simulink model "Autoex"  (Simulink 6.5)
settings: Solver=ode23t  StartTime=0.0  StopTime=10  RelTol=1e-3
undefined symbols (not defined in the file): powergui
libraries: powerlib x10, powerlib_extras x1
settings Model: Creator=RS  LastModifiedBy=RS

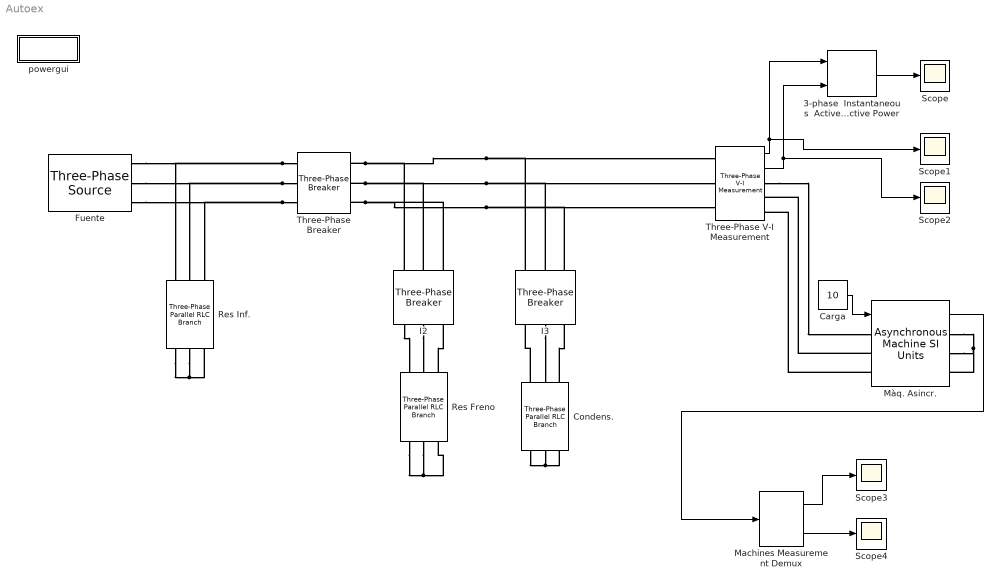
== system Autoex ==
  3-phase  Instantaneous  Active & Reactive Power : powerlib_extras/Measurements/3-phase  Instantaneous  Active & Reactive Power  DialogController=PMDialogs.PMDefaultMaskDlg  SystemSampleTime=-1
  Carga : Constant  Value=10  OutDataType=sfix(16)  ConRadixGroup=Use specified scaling  OutScaling=2^0  SampleTime=inf  FramePeriod=inf
  Condens. : powerlib/Elements/Three-Phase Parallel RLC Branch  Orientation=down  DialogController=PMDialogs.PMDefaultMaskDlg  PhysicalDomain=powersysdomain  SubClassName=unknown  LeftPortType=p1  RightPortType=p1  LConnTagsString=A|B|C  RConnTagsString=A|B|C  BranchType=C  Resistance=1  Inductance=1e-3  Capacitance=96.5e-6  Measurements=None
  Fuente : powerlib/Electrical Sources/Three-Phase Source  DialogController=PMDialogs.PMDefaultMaskDlg  SystemSampleTime=-1  Voltage=380  PhaseAngle=0  Frequency=50  InternalConnection=Yg  SpecifyImpedance=off  Resistance=0.0001  Inductance=0.0001  ShortCircuitLevel=100e6  BaseVoltage=25e3  XRratio=7
  I2 : powerlib/Elements/Three-Phase Breaker  Orientation=up  DialogController=PMDialogs.PMDefaultMaskDlg  SystemSampleTime=-1  InitialState=open  SwitchA=on  SwitchB=on  SwitchC=on  SwitchTimes=4  External=off  BreakerResistance=0.001  SnubberResistance=1e6  SnubberCapacitance=inf  Measurements=None
  I3 : powerlib/Elements/Three-Phase Breaker  Orientation=up  DialogController=PMDialogs.PMDefaultMaskDlg  SystemSampleTime=-1  InitialState=open  SwitchA=on  SwitchB=on  SwitchC=on  SwitchTimes=0  External=off  BreakerResistance=0.001  SnubberResistance=1e6  SnubberCapacitance=inf  Measurements=None
  Machines Measurement Demux : powerlib/Machines/Machines Measurement Demux  DialogController=PMDialogs.PMDefaultMaskDlg  SystemSampleTime=-1  machType=Asynchronous  ssm1=on  ssm2=on  ssm3=on  ssm4=on  ssm5=on  ssm6=on  sm1=off  sm2=off  sm3=off  sm4=off  sm5=off  sm6=off  sm7=off  sm8=on  sm9=off  sm10=off  sm11=off  sm115=off  sm12=off  sm13=off  sm14=off  asm1=off  asm2=off  asm3=off  asm4=off  asm5=off  asm6=off  asm7=off  asm8=off  asm9=on  asm10=on  asm11=off  pmsm1=on  pmsm2=on  pmsm3=on  pmsm4=off  pmsm5=on  pmsm6=on  pmsm7=on  lastType=1
  Màq. Asincr. : powerlib/Machines/Asynchronous Machine SI Units  DialogController=PMDialogs.PMDefaultMaskDlg  SystemSampleTime=-1  PresetModel=No  MechanicalLoad=Torque Tm  ShowDetailedParameters=on  RotorType=Wound  ReferenceFrame=Stationary  NominalParameters="[6.5*746   380   50]"  Stator="[0.63  0.00496]"  Rotor="[1.094   0.00496]"  Lm=0.105  Mechanical="[0.041   0   2]"  PolePairs=2  InitialConditions="[ 0,0   0,0,0   0,0,0 ]"  Units=1  LoadFlowParameters=0  SimulateSaturation=off  Saturation=[9.9249,19.6672,38.0377,51.3988,69.2824,105.1337,152.5532,214.2421,303.1917;230, 322, 414, 460, 506, 552, 598, 644, 690]
  Res Freno : powerlib/Elements/Three-Phase Parallel RLC Branch  Orientation=down  DialogController=PMDialogs.PMDefaultMaskDlg  PhysicalDomain=powersysdomain  SubClassName=unknown  LeftPortType=p1  RightPortType=p1  LConnTagsString=A|B|C  RConnTagsString=A|B|C  BranchType=R  Resistance=50  Inductance=1e-3  Capacitance=1e-6  Measurements=None
  Res Inf. : powerlib/Elements/Three-Phase Parallel RLC Branch  Orientation=down  DialogController=PMDialogs.PMDefaultMaskDlg  PhysicalDomain=powersysdomain  SubClassName=unknown  LeftPortType=p1  RightPortType=p1  LConnTagsString=A|B|C  RConnTagsString=A|B|C  BranchType=R  Resistance=1000000  Inductance=1e-3  Capacitance=1e-6  Measurements=None
  Scope{,1..4} (5 alike) : Scope
      Scope settings: MaxDataPoints=10000000  SampleInput=on  SampleTime=10e-6
      Scope1 settings: YMin=-1500  YMax=1500  MaxDataPoints=10000000  SampleInput=on  SampleTime=10e-6
      Scope2 settings: SaveName=ScopeData2  MaxDataPoints=10000000  SampleInput=on  SampleTime=10e-6
      Scope3 settings: SaveName=ScopeData3  MaxDataPoints=10000000  SampleInput=on  SampleTime=10e-6
      Scope4 settings: SaveName=ScopeData4  MaxDataPoints=10000000  SampleInput=on  SampleTime=10e-6
  Three-Phase V-I Measurement : powerlib/Measurements/Three-Phase V-I Measurement  DialogController=PMDialogs.PMDefaultMaskDlg  SystemSampleTime=-1  VoltageMeasurement=phase-to-ground  SetLabelV=off  LabelV=Vabc  Vpu=off  CurrentMeasurement=yes  SetLabelI=off  LabelI=Iabc  Ipu=off  Pbase=100e6  Vbase=500e3  OutputType=Complex  PhasorSimulation=off  PSBequivalent=0
  Three-Phase Breaker : powerlib/Elements/Three-Phase Breaker  DialogController=PMDialogs.PMDefaultMaskDlg  SystemSampleTime=-1  InitialState=closed  SwitchA=on  SwitchB=on  SwitchC=on  SwitchTimes=0  External=off  BreakerResistance=0.001  SnubberResistance=1e6  SnubberCapacitance=inf  Measurements=None
  powergui : Subsystem  AncestorBlock=powerlib/powergui  InitFcn=powergui( 'InitFcn_Callback' , gcb , 0 , [ ] );  mask(PSB option menu block){SimulationMode=Continuous, SampleTime=50e-6, echomessages=off, RestoreLinks=warning, x0status=blocks, Frange=[0:2:500], Ylog=off, Xlog=on, ShowGrid=off, save=off, variable=ZData, structure=, ZoomFFT=on, StartTime=0.0, cycles=1, DisplayStyle=1, fundamental=60, FreqAxis=off, MaxFrequency=1000, frequencyindice=50, frequencyindicesteady=1, RmsSteady=1, display=off, Ts=0, frequency=60, methode=off, HookPort=off, Interpol=off}
      mask prompts: SimulationMode "Simulation mode"; SampleTime "Sample time Ts (when simulation mode is Discrete) (s)"; echomessages "Echo  Messages"; RestoreLinks "Restore disabled links"; x0status "Initial electrical states status"; Frange "Impedance tool: Frequency Range"; Ylog "Impedance tool: Log impedance"; Xlog "Impedance tool: log Frequency"; ShowGrid "Impedance tool: grid"; save "Impedance tool: Save Data To Workspace"; variable "Impedance tool: Variable Name"; structure "Structure Name (PSBFFTSCOPE)"; ZoomFFT "ZoomFFT (PSBFFTSCOPE)"; StartTime "Start Time (PSBFFTSCOPE)"; cycles "Cycles (PSBFFTSCOPE)"; DisplayStyle "Display style (PSBFFTSCOPE)"; fundamental "Fundamental (PSBFFTSCOPE)"; FreqAxis "Frequency Axis (PSBFFTSCOPE)"; MaxFrequency "Max Frequency (PSBFFTSCOPE)"; frequencyindice "Load flow frequency (Hz)"; frequencyindicesteady "Frequency indice (STEADYSTATE)"; RmsSteady "RMS display (STEADYSTATE)"; display "Display Results"; Ts "OBSOLETE 1"; frequency "Phasor frequency (Hz)"; methode "Phasor simulation"; HookPort "Hook port"; Interpol "Interpolate"
      mask init:
      | powerlibroot = which('powersysdomain');
      | PSBroot = powerlibroot(1:end-16);
      | %
      | switch SimulationMode
      | 	case 1
      | 		message=sprintf('Continuous');
      | 	case 2
      |         SampleTimeeval=evalin('base',SampleTime,'NaN');
      |         if isnan(SampleTimeeval)
      |             message=sprintf('Warning !!,\nUndefined sample time');
      |         else
      |             message=sprintf('Discrete,\nTs = %.4g s.',SampleTimeeval);
      |         end
      | 	case 3
      | 		message=sprintf('Phasors');
      | end
      | if strcmp(bdroot,'powerlib')
      |   message='powergui';
      | end
      | power_initmask();
      settings: CopyFcn=powergui( 'Copy_Callback' , gcb , 0 , [ ] );  ModelCloseFcn=powergui( 'CloseButton_Callback' , gcb , [ ] , [ ] );  PreSaveFcn=powergui( 'CloseButton_Callback' , gcb , [ ] , [ ] );  NameChangeFcn=powergui( 'NameChangeFcn_Callback' , gcb , 0 , [ ] );
      settings: DeleteFcn=|
      | powergui( 'Copy_Callback' , gcb , 1 , [ ] );
      | powergui( 'CloseButton_Callback' , gcb , [ ] , [ ] );
      settings: OpenFcn=|
      | if (power_openblockproxy ('secondary'))
      | powergui(gcb,'PM')
      | end;
      mask Help: web(psbhelp)
      mask StyleString: popup(Continuous|Discrete|Phasor),edit,checkbox,popup(yes|warning|no),popup(blocks|steady|zero),edit,checkbox,checkbox,checkbox,checkbox,edit,edit,checkbox,edit,edit,edit,edit,checkbox,edit,edit,edit,edit,checkbox,edit,edit,checkbox,checkbox,checkbox
      mask CallbackString: ||||||||||||||||||||||||||powergui('HookPort',[],[],gcb);|
      mask Display: disp(message)
  wires:
  Three-Phase V-I Measurement/1 -> 3-phase  Instantaneous  Active & Reactive Power/1, Scope1/1
  Three-Phase V-I Measurement/2 -> 3-phase  Instantaneous  Active & Reactive Power/2, Scope2/1
  Màq. Asincr./1 -> Machines Measurement Demux/1
  Carga/1 -> Màq. Asincr./1
  3-phase  Instantaneous  Active & Reactive Power/1 -> Scope/1
  Machines Measurement Demux/1 -> Scope3/1
  Machines Measurement Demux/2 -> Scope4/1
  connections:
  Three-Phase Breaker/RConn2 -- I2/RConn2 -- Three-Phase V-I Measurement/LConn2 -- I3/RConn2
  Three-Phase Breaker/RConn1 -- I2/RConn1 -- Three-Phase V-I Measurement/LConn1 -- I3/RConn1
  Three-Phase Breaker/RConn3 -- I2/RConn3 -- Three-Phase V-I Measurement/LConn3 -- I3/RConn3
  I2/LConn1 -- Res Freno/LConn1
  I2/LConn2 -- Res Freno/LConn2
  Res Freno/LConn3 -- I2/LConn3
  I3/LConn2 -- Condens./LConn2
  Condens./LConn1 -- I3/LConn1
  Condens./LConn3 -- I3/LConn3
  Three-Phase V-I Measurement/RConn1 -- Màq. Asincr./LConn1
  Màq. Asincr./LConn2 -- Three-Phase V-I Measurement/RConn2
  Màq. Asincr./LConn3 -- Three-Phase V-I Measurement/RConn3
  Three-Phase Breaker/LConn1 -- Fuente/RConn1 -- Res Inf./LConn1
  Three-Phase Breaker/LConn2 -- Fuente/RConn2 -- Res Inf./LConn2
  Three-Phase Breaker/LConn3 -- Fuente/RConn3 -- Res Inf./LConn3
  Res Inf./RConn1 -- Res Inf./RConn3 -- Res Inf./RConn2
  Res Freno/RConn1 -- Res Freno/RConn3 -- Res Freno/RConn2
  Condens./RConn1 -- Condens./RConn3 -- Condens./RConn2
  Màq. Asincr./RConn1 -- Màq. Asincr./RConn3 -- Màq. Asincr./RConn2

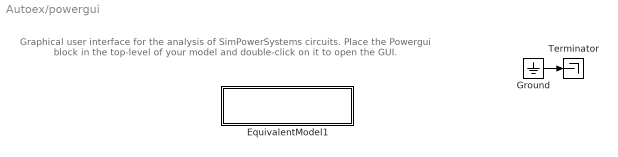
== system Autoex/powergui ==
  note: Graphical user interface for the analysis of  SimPowerSystems circuits.
      | Place the Powergui block in the top-level of your model and double-click
      | on it to open the GUI.
  EquivalentModel1 : Subsystem
      mask init:
      | SPS = get_param(gcbh,'UserData');
      | if isempty(SPS)
      |     A=0;
      |     B=0;
      |     C=0;
      |     D=0;
      |     x0=0;
      |     SwitchResistance=1;
      |     SwitchType=1;
      |     SwitchGateInitialValue=1;
      |     OutputsToResetToZero=1;
      | else
      | 	A=SPS.A;
      |     B=SPS.B;
      |     C=SPS.C;
      |     D=SPS.D;
      |     x0=SPS.x0;
      |     SwitchResistance=SPS.SwitchResistance;
      |     SwitchType=SPS.SwitchType;
      |     SwitchGateInitialValue=SPS.SwitchGateInitialValue;
      |     OutputsToResetToZero=SPS.YSwitchCurrent;
      | end
      mask Display:
      | color('blue')
      | disp('EQUIVALENT CIRCUIT')
  Ground : Ground
  Terminator : Terminator
  wires:
  Ground/1 -> Terminator/1

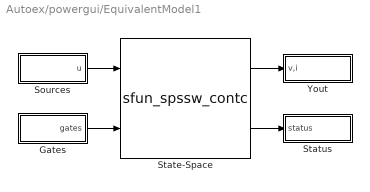
== system Autoex/powergui/EquivalentModel1 ==
  Gates : Subsystem
  Sources : Subsystem
  State-Space : S-Function  FunctionName=sfun_spssw_contc  Parameters=A, B, C, D, x0, SwitchResistance ,SwitchType, SwitchGateInitialValue, OutputsToResetToZero
  Status : Subsystem
  Yout : Subsystem
  wires:
  Gates/1(gates) -> State-Space/2
  Sources/1(u) -> State-Space/1
  State-Space/2 -> Status/1(status)
  State-Space/1 -> Yout/1(v,i)

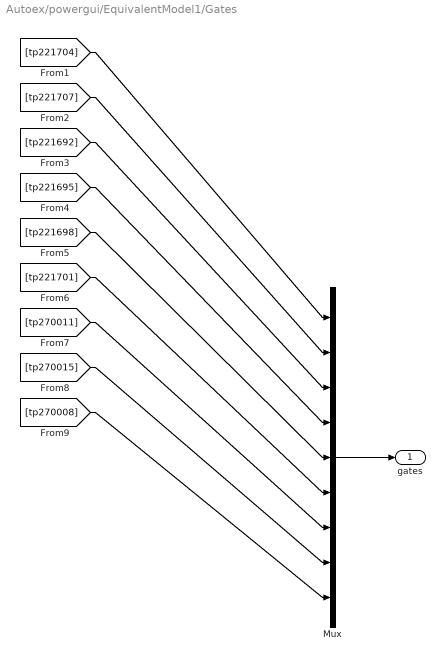
== system Autoex/powergui/EquivalentModel1/Gates ==
  Mux : Mux  Inputs=[1 1 1 1 1 1 1 1 1]
  gates : Outport
  wires:
  Mux/1 -> gates/1
  [tp221704] -> Mux/1
  [tp221707] -> Mux/2
  [tp221692] -> Mux/3
  [tp221695] -> Mux/4
  [tp221698] -> Mux/5
  [tp221701] -> Mux/6
  [tp270011] -> Mux/7
  [tp270015] -> Mux/8
  [tp270008] -> Mux/9

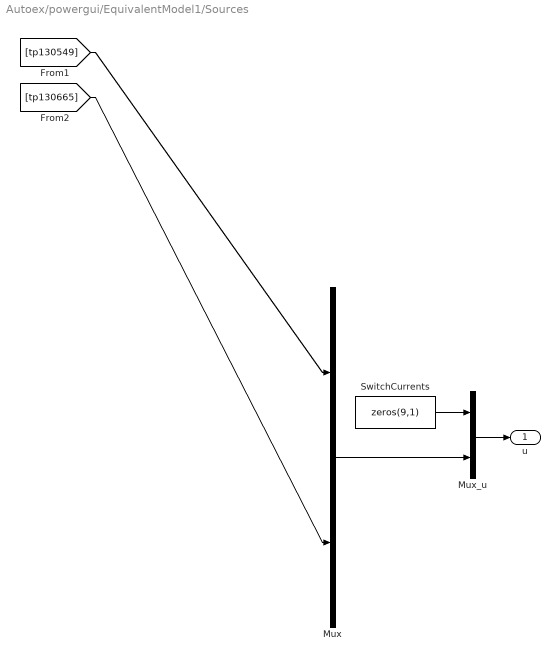
== system Autoex/powergui/EquivalentModel1/Sources ==
  Mux : Mux  Inputs=[4 3]
  Mux_u : Mux  Inputs=[9 7]
  SwitchCurrents : Constant  Value=zeros(9,1)  OutDataType=sfix(16)  ConRadixGroup=Use specified scaling  OutScaling=2^0  SampleTime=inf  FramePeriod=inf
  u : Outport
  wires:
  Mux/1 -> Mux_u/2
  SwitchCurrents/1 -> Mux_u/1
  Mux_u/1 -> u/1
  [tp130549] -> Mux/1
  [tp130665] -> Mux/2

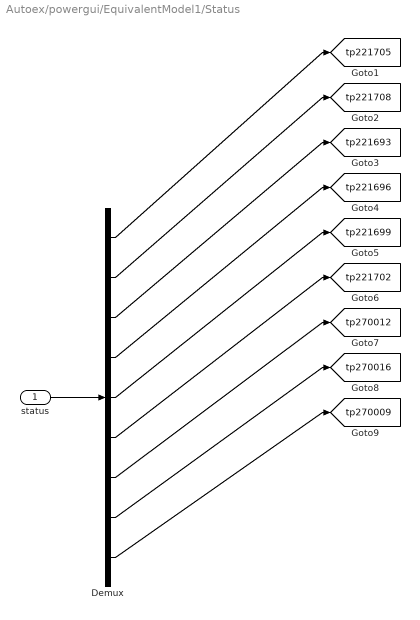
== system Autoex/powergui/EquivalentModel1/Status ==
  status : Inport
  Demux : Demux  Outputs=[1 1 1 1 1 1 1 1 1]
  tag scope: tp221693=global, tp221696=global, tp221699=global, tp221702=global, tp221705=global, tp221708=global, tp270009=global, tp270012=global, tp270016=global
  wires:
  status/1 -> Demux/1
  Demux/1 -> [tp221705]
  Demux/2 -> [tp221708]
  Demux/3 -> [tp221693]
  Demux/4 -> [tp221696]
  Demux/5 -> [tp221699]
  Demux/6 -> [tp221702]
  Demux/7 -> [tp270012]
  Demux/8 -> [tp270016]
  Demux/9 -> [tp270009]

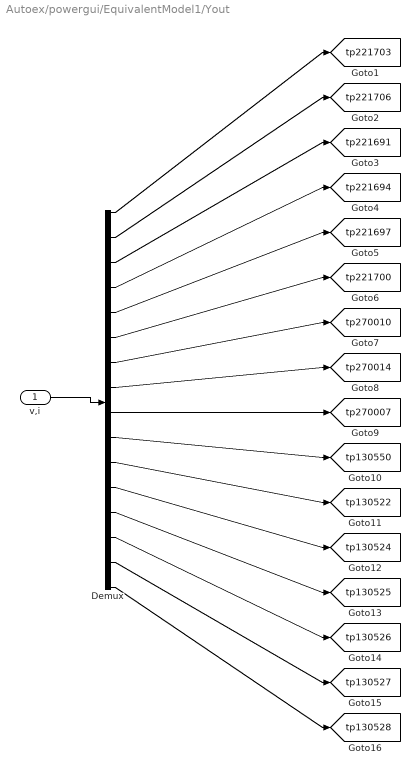
== system Autoex/powergui/EquivalentModel1/Yout ==
  v,i : Inport
  Demux : Demux  Outputs=[1 1 1 1 1 1 1 1 1 4 1 1 1 1 1 1]
  tag scope: tp130522=global, tp130524=global, tp130525=global, tp130526=global, tp130527=global, tp130528=global, tp130550=global, tp221691=global, tp221694=global, tp221697=global, tp221700=global, tp221703=global, tp221706=global, tp270007=global, tp270010=global, tp270014=global
  wires:
  v,i/1 -> Demux/1
  Demux/1 -> [tp221703]
  Demux/2 -> [tp221706]
  Demux/3 -> [tp221691]
  Demux/4 -> [tp221694]
  Demux/5 -> [tp221697]
  Demux/6 -> [tp221700]
  Demux/7 -> [tp270010]
  Demux/8 -> [tp270014]
  Demux/9 -> [tp270007]
  Demux/10 -> [tp130550]
  Demux/11 -> [tp130522]
  Demux/12 -> [tp130524]
  Demux/13 -> [tp130525]
  Demux/14 -> [tp130526]
  Demux/15 -> [tp130527]
  Demux/16 -> [tp130528]
